simulink model "vector_control_induction_machine"  (Simulink 7.3)
settings: Solver=ode45  StartTime=0.0  StopTime=2  RelTol=1e-3
InitFcn:
  | % Processor selection for I/O assignment
  | % The chosen Target in the Coder Options window must match the selected MCU.
  | % Set the variable 'type_evm' to the following strings to choose a specific target:
  | 
  |   type_evm = 'TI28069';    % TI28069 Piccolo Launchpad
  | % type_evm = 'TI28377S';   % TI28377S Delfino Launchpad
  | % type_evm = 'TI28379LP';  % TI28379D Delfino Launchpad
  | % type_evm = 'TI280049C';  % TI280049C Piccolo Launchpad
  | % type_evm = 'TI28335';    % TI28335 Delfino Controlcard
  | % type_evm = 'TI28379CC';  % TI28379D Delfino Controlcard
  | % type_evm = 'TI28388D';   % TI28388D Controlcard
  | 
  | % -- IMPORTANT --
  | % For TI280049 Launchpad, make sure on the Launchpad switches S6, S8, S4 are set as 1, i.e. pushed to the dot side.
  | % And switch S3.1 also set as 1, i.e. pushed to BP (bypass) side.
  | 
  | 
  | % Configure I/O based on processor
  | switch (type_evm)
  | 	case 'TI28069'
  | 	% Configuration for TI28069 Launchpad
  | 	% On the Plant side
  | 		AO_RTBox_Vdc = 3;
  | 		AO_RTBox_Is = [0:2];
  | 		ENC_RTBox_A = 6;
  | 		ENC_RTBox_B = 7;
  | 		ENC_RTBox_I = 23;
  | 		PWMCAP_RTBox_sw = [0:5];
  | 		DI_RTBox_Eni = 29;
  | 		DO_RTBox_Eno = 4;
  | 		DI_RTBox_Tzi = 28;
  | 		DO_RTBox_Tzo = 2;
  | 		DI_RTBox_Power = 22;
  | 
  | 	% On the MCU side
  | 		ADC_DSP_ADC = [7,9,2,10];
  | 		eQEP_DSP_eQEP = 1;
  | 		QEP_DSP_QEP = [50,51,53];
  | 		PWM_DSP_PWM = [1,2,3];
  | 		DO_DSP_LED = 34;
  | 		DI_DSP_En = 13;
  | 		TZ_DSP_Tz1 = 12;
  | 		TZ_DSP_Tz1_mode = 3;
  | 		TZ_DSP_Tz2 = nan;
  | 		TZ_DSP_Tz2_mode = 1;
  | 		PWR_DSP_GPIO = 27;
  | 
  | 		SCI_DSP = [28, 29];
  | 		AO_Factor = 1;
  | 		AO_Vmax = 3.3;
  | 		ADC_Vmax = 3.3;
  | 
  | 	case 'TI28377S'
  | 	% Configuration for TI28377S Launchpad
  | 	% On the Plant side
  | 		AO_RTBox_Vdc = 12;
  | 		AO_RTBox_Is = [4,6,9]; % DSP ADCINA0, A1, A2, A3
  | 		ENC_RTBox_A = 4;
  | 		ENC_RTBox_B = 5;
  | 		ENC_RTBox_I = 22;
  | 		PWMCAP_RTBox_sw = [2,3,4,5,20,21];
  | 		DI_RTBox_Eni = 29;
  | 		DO_RTBox_Eno = 6;
  | 		DI_RTBox_Tzi = 28;
  | 		DO_RTBox_Tzo = 7;
  | 		DI_RTBox_Power = 26;
  | 
  | 	% On the MCU side
  | 		ADC_DSP_ADC = [0,1,2,3];
  | 		eQEP_DSP_eQEP = 1;
  | 		QEP_DSP_QEP = [20,21,99];
  | 		PWM_DSP_PWM = [8,9,10];
  | 		DO_DSP_LED = 12;
  | 		DI_DSP_En = 72;
  | 		TZ_DSP_Tz1 = 73;
  | 		TZ_DSP_Tz1_mode = 3;
  | 		TZ_DSP_Tz2 = nan;
  | 		TZ_DSP_Tz2_mode = 1;
  | 		PWR_DSP_GPIO = 43;
  | 
  | 		SCI_DSP = [85, 84];
  | 		AO_Factor = 1;
  | 		AO_Vmax = 3.3;
  | 		ADC_Vmax = 3.3;
  | 
  | 	case 'TI28379LP'
  | 	% Configuration for TI28379LP Launchpad
  | 	% On the Plant side
  | 		AO_RTBox_Vdc = 14;
  | 		AO_RTBox_Is = [3,7,11];
  | 		ENC_RTBox_A = 4;
  | 		ENC_RTBox_B = 24;
  | 		ENC_RTBox_I = 22;
  | 		PWMCAP_RTBox_sw = [0:5];
  | 		DI_RTBox_Eni = 29;
  | 		DO_RTBox_Eno = 6;
  | 		DI_RTBox_Tzi = 28;
  | 		DO_RTBox_Tzo = 7;
  | 		DI_RTBox_Power = 22;
  | 
  | 	% On the MCU side
  | 		ADC_DSP_ADC = [3,0,5,4];
  | 		eQEP_DSP_eQEP = 2;
  | 		QEP_DSP_QEP = [24,25,26];
  | 		PWM_DSP_PWM = [1,2,3];
  | 		DO_DSP_LED = 34;
  | 		DI_DSP_En = 124;
  | 		TZ_DSP_Tz1 = 125;
  | 		TZ_DSP_Tz1_mode = 3;
  | 		TZ_DSP_Tz2 = nan;
  | 		TZ_DSP_Tz2_mode = 1;
  | 		PWR_DSP_GPIO = 66;
  | 
  | 		SCI_DSP = [43, 42];
  | 		AO_Factor = 1;
  | 		AO_Vmax = 3.3;
  | 		ADC_Vmax = 3.3;
  | 
  | 	case 'TI280049C'
  | 	% Configuration for TI280049C Launchpad
  | 	% On the Plant side
  | 		AO_RTBox_Vdc = 6;
  | 		AO_RTBox_Is = [7,14,8];
  | 		ENC_RTBox_A = 16;
  | 		ENC_RTBox_B = 17;
  | 		ENC_RTBox_I = 3;
  | 		PWMCAP_RTBox_sw = [0:5];
  | 		DI_RTBox_Eni = 29;
  | 		DO_RTBox_Eno = 4;
  | 		DI_RTBox_Tzi = 28;
  | 		DO_RTBox_Tzo = 5;
  | 		DI_RTBox_Power = 24;
  | 
  | 	% On the MCU side
  | % -- IMPORTANT --
  | % For TI280049 Launchpad, make sure on the Launchpad switches S6, S8, S4 are set as 1, i.e. pushed to the dot side.
  | % And switch S3.1 also set as 1, i.e. pushed to BP (bypass) side.
  | 		ADC_DSP_ADC = [1,3,6,9];
  | 		eQEP_DSP_eQEP = 1;
  | 		QEP_DSP_QEP = [28,29,59];
  | 		PWM_DSP_PWM = [6,5,3];
  | 		DO_DSP_LED = 34;
  | 		DI_DSP_En = 58;
  | 		TZ_DSP_Tz1 = 30;
  | 		TZ_DSP_Tz1_mode = 3;
  | 		TZ_DSP_Tz2 = nan;
  | 		TZ_DSP_Tz2_mode = 1;
  | 		PWR_DSP_GPIO = 56;
  | 
  | 		SCI_DSP = [35, 37]; %Cannot use [28,29] since they are already used for eQEP1A-1B.
  | 		AO_Factor = 1;
  | 		AO_Vmax = 3.3;
  | 		ADC_Vmax = 3.3;
  | 
  | 	case 'TI28335'
  | 	% Configuration for TI28335 Controlcard
  | 	% On the Plant side
  | 		AO_RTBox_Vdc = 9;
  | 		AO_RTBox_Is = [15,13,11];
  | 		ENC_RTBox_A = 2;
  | 		ENC_RTBox_B = 3;
  | 		ENC_RTBox_I = 1;
  | 		PWMCAP_RTBox_sw = [17,16,19,18,21,20];
  | 		DI_RTBox_Eni = 29;
  | 		DO_RTBox_Eno = 6;
  | 		DI_RTBox_Tzi = 28;
  | 		DO_RTBox_Tzo = 0;
  | 		DI_RTBox_Power = 27;
  | 
  | 	% On the MCU side
  | 		ADC_DSP_ADC = [0,1,2,3];
  | 		eQEP_DSP_eQEP = 1;
  | 		QEP_DSP_QEP = [20,21,23];
  | 		eQEP_DSP_eQEP = 1;
  | 		PWM_DSP_PWM = [1,2,3];
  | 		DO_DSP_LED = 34;
  | 		DI_DSP_En = 24;
  | 		TZ_DSP_Tz1 = 12;
  | 		TZ_DSP_Tz1_mode = 1;
  | 		TZ_DSP_Tz2 = 13;
  | 		TZ_DSP_Tz2_mode = 3;
  | 		PWR_DSP_GPIO = 10;
  | 
  | 		SCI_DSP = [28, 29];
  | 		AO_Factor = 1.54;
  | 		AO_Vmax = 5;
  | 		ADC_Vmax = 3;
  | 
  | 	case 'TI28379CC'
  | 	% Configuration for TI28379D Controlcard
  | 	% On the Plant side
  | 		AO_RTBox_Vdc = 9;
  | 		AO_RTBox_Is = [15,13,11];
  | 		ENC_RTBox_A = 13;
  | 		ENC_RTBox_B = 14;
  | 		ENC_RTBox_I = 26;
  | 		PWMCAP_RTBox_sw = [0,1,2,3,4,5];
  | 		DI_RTBox_Eni = 29;
  | 		DO_RTBox_Eno = 21;
  | 		DI_RTBox_Tzi = 28;
  | 		DO_RTBox_Tzo = 20;
  | 		DI_RTBox_Power = 14;
  | 
  | 		% On the MCU side
  | 		ADC_DSP_ADC = [0,1,2,3];
  | 		eQEP_DSP_eQEP = 1;
  | 		QEP_DSP_QEP = [20,21,23];
  | 		PWM_DSP_PWM = [1,2,3];
  | 		DO_DSP_LED = 34;
  | 		DI_DSP_En = 40;
  | 		TZ_DSP_Tz1 = 41;
  | 		TZ_DSP_Tz1_mode = 3;
  | 		TZ_DSP_Tz2_mode = 1;
  | 		PWR_DSP_GPIO = 39;
  | 
  | 		SCI_DSP = [28, 29];
  | 		AO_Factor = 1.54; % breakout board scaling 6.8k/4.42k
  | 		AO_Vmax = 5.0;
  | 		ADC_Vmax = 3.0; % ADC reference
  | 
  | 	case 'TI28388D'
  | 	% Configuration for TI28388D Controlcard
  | 	% On the Plant side
  | 		AO_RTBox_Vdc = 9;
  | 		AO_RTBox_Is = [15,13,11];
  | 		ENC_RTBox_A = 13;
  | 		ENC_RTBox_B = 14;
  | 		ENC_RTBox_I = 26;
  | 		PWMCAP_RTBox_sw = [0,1,2,3,4,5];
  | 		DI_RTBox_Eni = 29;
  | 		DO_RTBox_Eno = 21;
  | 		DI_RTBox_Tzi = 28;
  | 		DO_RTBox_Tzo = 20;
  | 		DI_RTBox_Power = 14;
  | 
  | 		% On the MCU side
  | 		ADC_DSP_ADC = [0,1,2,3];
  | 		eQEP_DSP_eQEP = 1;
  | 		QEP_DSP_QEP = [20,21,23];
  | 		PWM_DSP_PWM = [1,2,3];
  | 		DO_DSP_LED = 34;
  | 		DI_DSP_En = 40;
  | 		TZ_DSP_Tz1 = 41;
  | 		TZ_DSP_Tz1_mode = 3;
  | 		TZ_DSP_Tz2_mode = 1;
  | 		PWR_DSP_GPIO = 39;
  | 
  | 		SCI_DSP = [28, 29];
  | 		AO_Factor = 1.54; % breakout board scaling 6.8k/4.42k
  | 		AO_Vmax = 5.0;
  | 		ADC_Vmax = 3.0; % ADC reference
  | 
  | 
  | 	otherwise
  | 	error('Unknown evaluation module selection, please choose either ''TI28069'', ''TI28377S'', ''TI28379LP'', ''TI280049C'', ''TI28335'', ''TI28379CC'' or ''TI28388D''.')
  | end
  | 
  | 
  | % Induction Machine
  | Rs = 0.1062;
  | Rr = 0.0764;
  | Lls = 0.2145/(2*pi*60);
  | Llr = Lls;
  | Lm = 5.834/(2*pi*60);
  | Lr = Lm + Llr;
  | Ls = Lm + Lls;
  | p = 2;
  | J = 2.8;
  | F = 0;
  | 
  | % Rotor flux orientation
  | k = Lm/sqrt(Lr*Ls);
  | sigma = 1 - k^2;
  | Lsigma = sigma*Ls;
  | Tr = Lr/Rr;
  | LM = Lm*(Lm/Lr);
  | RR = Rr*(Lm/Lr)^2;
  | 
  | % Converter
  | Vdc = 400;
  | fsw = 10e3;
  | 
  | % PI controller
  | Rtot = Rs + Rr*(Lm/Lr)^2;
  | 
  | Lf_PI = Lsigma;
  | Rf_PI = Rtot;
  | K_plant = 1/Rf_PI;
  | T_plant = Lf_PI/Rf_PI;
  | 
  | Kpe = 1;
  | Tsw = 1/fsw;
  | Tpe = Tsw*1.5;
  | 
  | type_PI = 2;
  | 
  | % PI design: Maximum Gain
  | PM_PI = 50;
  | wc_PI = (90-PM_PI)/180*pi/Tpe;
  | Kp_PI = wc_PI*Lf_PI/Kpe;
  | Ti_PI = 10*Kpe/(wc_PI^2*Lf_PI);
  | Ki_PI = 1/Ti_PI;
  | Kbc_PI = Ki_PI/Kp_PI;
  | 
  | % HIL simulation
  | Ts_plant = 5e-6;
  | Ts_controller = 1/fsw;
  | 
  | % Scaling
  | Vdc_scl = ADC_Vmax/Vdc;
  | Is_scl = ADC_Vmax/2/300;
  | Is_ofs = ADC_Vmax/2;
undefined symbols (not defined in the file): plecs
settings Model: Creator=kris  LastModifiedBy=manaswini  ExtModeTrigMode=oneshot  ExtModeArmWhenConnect=off  ExtModeAutoUpdateStatusClock=off
settings DataIOCC: LimitDataPoints=off  ReturnWorkspaceOutputs=off  SignalLoggingName=sigsOut
settings OptimizationCC: BooleanDataType=off  ExpressionDepthLimit=128  InitFltsAndDblsToZero=on
settings DebuggingCC: SaveWithParameterizedLinksMsg=none  SignalResolutionControl=TryResolveAllWithWarning  SolverPrmCheckMsg=none  MultiTaskDSMMsg=warning  MultiTaskCondExecSysMsg=none  FcnCallInpInsideContextMsg=Enable All  StrictBusMsg=ErrorLevel1
settings HardwareCC: TargetHWDeviceType=32-bit Generic  TargetUnknown=on  ProdEqTarget=off
settings RTWCC: IncludeERTFirstTime=on
settings CodeAppCC: CustomSymbolStrType=$N$R$M_T
settings GRTTargetCC: TargetFcnLib=ansi_tfl_tmw.mat  TargetFunctionLibrary=C89/C90 (ANSI)  ModelReferenceCompliant=off

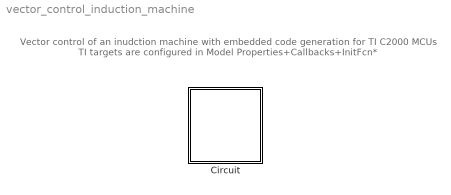
== system vector_control_induction_machine ==
  note: Vector control of an inudction machine
      | with embedded code generation for TI C2000 MCUs
      | TI targets are configured in Model Properties+Callbacks+InitFcn*
  Circuit : Subsystem  LoadFcn=plecs('sl', 200);  InitFcn=plecs('sl', 214);  StartFcn=plecs('sl', 208);  StopFcn=plecs('sl', 209);  ClipboardFcn=plecs('sl', 212, 30);  mask(PlecsCircuit){PLECSData=<binary blob, 28632 chars, not shown>}
      mask prompts: PLECSData "PLECS Data (Do not delete or modify!)"
      mask help: Drag this block into a Simulink model to create a new electrical circuit.
      mask init:
      | % PLACE CUSTOM INITIALIZATIONS ABOVE
      | % DO NOT REMOVE
      | plecs('sl', 215);
      | % DO NOT REMOVE
      settings: CopyFcn=plecs('sl', 203);  DeleteFcn=plecs('sl', 205);  UndoDeleteFcn=plecs('sl', 206);  PreSaveFcn=plecs('sl', 211);  PostSaveFcn=plecs('sl', 201);  NameChangeFcn=plecs('sl', 210);  DestroyFcn=plecs('sl', 207);  PreCopyFcn=plecs('sl', 216);  OpenFcn=plecs('sl', 202);  ErrorFcn=plerrorfcn
      mask Display: disp('PLECS\nCircuit')

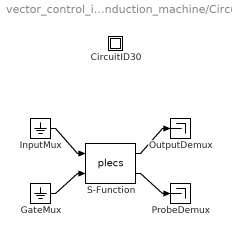
== system vector_control_induction_machine/Circuit ==
  " CircuitID30 " : Subsystem
  " GateMux " : Ground
  " InputMux " : Ground
  " OutputDemux " : Terminator
  " ProbeDemux " : Terminator
  " S-Function " : S-Function  FunctionName=plecs  EnableBusSupport=off
  wires:
  " InputMux "/1 -> " S-Function "/1
  " GateMux "/1 -> " S-Function "/2
  " S-Function "/1 -> " OutputDemux "/1
  " S-Function "/2 -> " ProbeDemux "/1

== system vector_control_induction_machine/Circuit/ CircuitID30  ==
